simulink model "inflowMatrix"  (R2018a)
settings: Solver=ode1  StartTime=0.0  StopTime=5  FixedStep=1/100  RelTol=1e-3
values from neighbouring files (symbols this model uses):
  s = (0.70:0.02:2.80)    [fy.m]
undefined symbols (not defined in the file or in its folder): deg, rad
libraries: aerolibconvert2 x6
settings Model: PauseTimes=25  Creator=ali  LastModifiedBy=ali

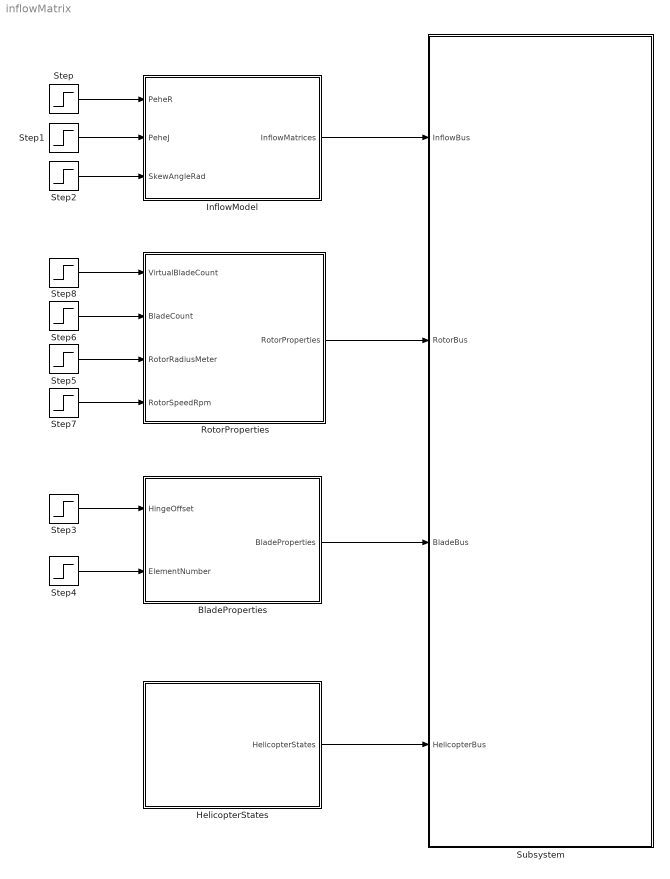
== system inflowMatrix ==
  BladeProperties : Subsystem  TreatAsAtomicUnit=on
  HelicopterStates : Subsystem  TreatAsAtomicUnit=on
  InflowModel : Subsystem  TreatAsAtomicUnit=on
  RotorProperties : Subsystem  TreatAsAtomicUnit=on
  Step : Step  Time=25  Before=2  After=4  SampleTime=0
  Step1 : Step  Time=25  Before=4  After=4  SampleTime=0
  Step2 : Step  Time=0.5  Before=0.0 * pi / 180  After=0.0 * pi / 180  SampleTime=0
  Step3 : Step  Time=0.5  Before=0.01  After=0.01  SampleTime=0
  Step4 : Step  Time=0.5  Before=10  After=10  SampleTime=0
  Step5 : Step  Time=0.5  Before=6  After=6  SampleTime=0
  Step6 : Step  Time=0.5  Before=4  After=4  SampleTime=0
  Step7 : Step  Time=0.5  Before=300  After=300  SampleTime=0
  Step8 : Step  Time=0.5  Before=8  After=8  SampleTime=0
  Subsystem : Subsystem  TreatAsAtomicUnit=on
  wires:
  Step/1 -> InflowModel/1(PeheR)
  Step1/1 -> InflowModel/2(PeheJ)
  Step2/1 -> InflowModel/3(SkewAngleRad)
  Step3/1 -> BladeProperties/1(HingeOffset)
  Step4/1 -> BladeProperties/2(ElementNumber)
  Step5/1 -> RotorProperties/3(RotorRadiusMeter)
  Step6/1 -> RotorProperties/2(BladeCount)
  Step7/1 -> RotorProperties/4(RotorSpeedRpm)
  RotorProperties/1(RotorProperties) -> Subsystem/2(RotorBus)
  BladeProperties/1(BladeProperties) -> Subsystem/3(BladeBus)
  InflowModel/1(InflowMatrices) -> Subsystem/1(InflowBus)
  HelicopterStates/1(HelicopterStates) -> Subsystem/4(HelicopterBus)
  Step8/1 -> RotorProperties/1(VirtualBladeCount)

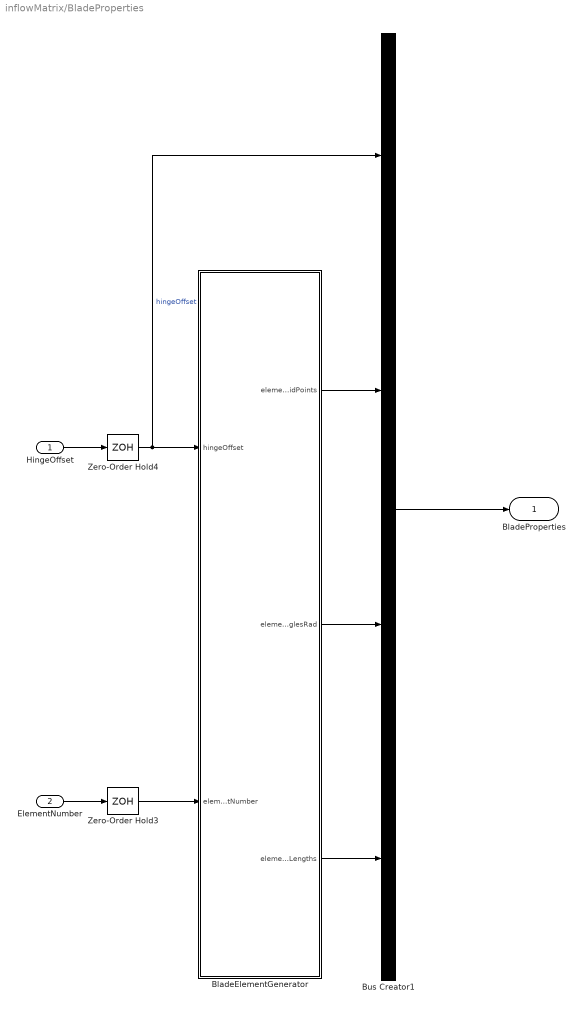
== system inflowMatrix/BladeProperties ==
  HingeOffset : Inport  OutDataTypeStr=double
  ElementNumber : Inport  Port=2  OutDataTypeStr=double
  BladeElementGenerator : MATLAB Function  TreatAsAtomicUnit=on
  Bus Creator1 : BusCreator  Inputs=4
  Zero-Order Hold3 : ZeroOrderHold  SampleTime=-1
  Zero-Order Hold4 : ZeroOrderHold  SampleTime=-1
  BladeProperties : Outport
  wires:
  Zero-Order Hold3/1 -> BladeElementGenerator/2(elementNumber)
  Zero-Order Hold4/1 -> Bus Creator1/1, BladeElementGenerator/1(hingeOffset)  "hingeOffset"
  HingeOffset/1 -> Zero-Order Hold4/1
  ElementNumber/1 -> Zero-Order Hold3/1
  Bus Creator1/1 -> BladeProperties/1
  BladeElementGenerator/1(elementMidPoints) -> Bus Creator1/2
  BladeElementGenerator/2(elementTwistAnglesRad) -> Bus Creator1/3
  BladeElementGenerator/3(elementChordLengths) -> Bus Creator1/4

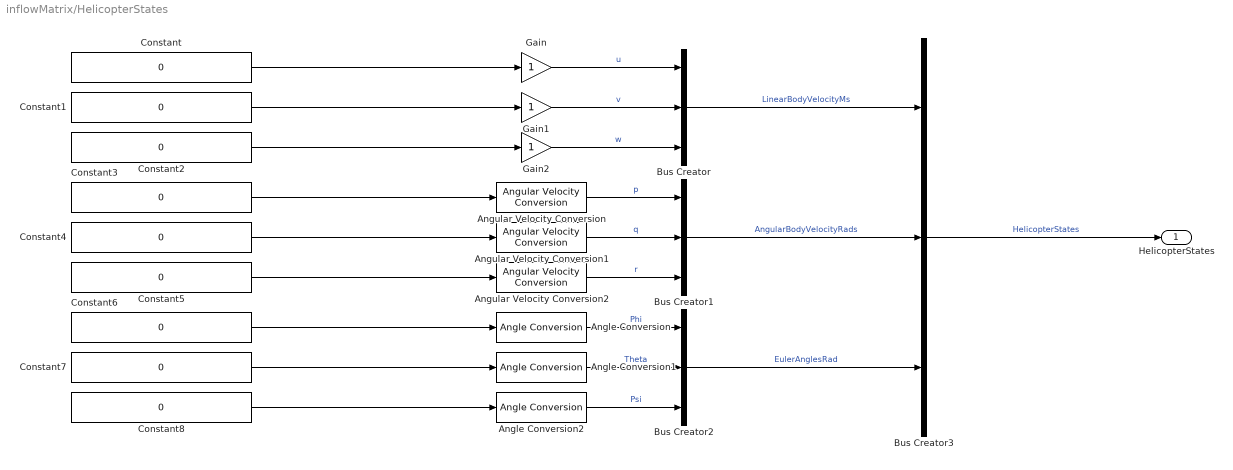
== system inflowMatrix/HelicopterStates ==
  Angle Conversion : aerolibconvert2/Angle Conversion  IU=deg  OU=rad
  Angle Conversion1 : aerolibconvert2/Angle Conversion  IU=deg  OU=rad
  Angle Conversion2 : aerolibconvert2/Angle Conversion  IU=deg  OU=rad
  Angular Velocity Conversion : aerolibconvert2/Angular Velocity Conversion  IU=deg/s  OU=rad/s
      settings: SourceProductName=Aerospace Blockset
  Angular Velocity Conversion1 : aerolibconvert2/Angular Velocity Conversion  IU=deg/s  OU=rad/s
      settings: SourceProductName=Aerospace Blockset
  Angular Velocity Conversion2 : aerolibconvert2/Angular Velocity Conversion  IU=deg/s  OU=rad/s
      settings: SourceProductName=Aerospace Blockset
  Bus Creator{,1..3} (4 alike) : BusCreator  Inputs=3
  Constant{,1..8} (9 alike) : Constant  Value=0
  Gain : Gain
  Gain1 : Gain
  Gain2 : Gain
  HelicopterStates : Outport
  wires:
  Bus Creator/1 -> Bus Creator3/1  "LinearBodyVelocityMs"
  Constant/1 -> Gain/1
  Constant1/1 -> Gain1/1
  Constant2/1 -> Gain2/1
  Gain/1 -> Bus Creator/1  "u"
  Gain1/1 -> Bus Creator/2  "v"
  Gain2/1 -> Bus Creator/3  "w"
  Constant3/1 -> Angular Velocity Conversion/1
  Constant4/1 -> Angular Velocity Conversion1/1
  Constant5/1 -> Angular Velocity Conversion2/1
  Angular Velocity Conversion/1 -> Bus Creator1/1  "p"
  Angular Velocity Conversion1/1 -> Bus Creator1/2  "q"
  Angular Velocity Conversion2/1 -> Bus Creator1/3  "r"
  Constant6/1 -> Angle Conversion/1
  Constant7/1 -> Angle Conversion1/1
  Constant8/1 -> Angle Conversion2/1
  Angle Conversion/1 -> Bus Creator2/1  "Phi"
  Angle Conversion1/1 -> Bus Creator2/2  "Theta"
  Angle Conversion2/1 -> Bus Creator2/3  "Psi"
  Bus Creator1/1 -> Bus Creator3/2  "AngularBodyVelocityRads"
  Bus Creator2/1 -> Bus Creator3/3  "EulerAnglesRad"
  Bus Creator3/1 -> HelicopterStates/1  "HelicopterStates"

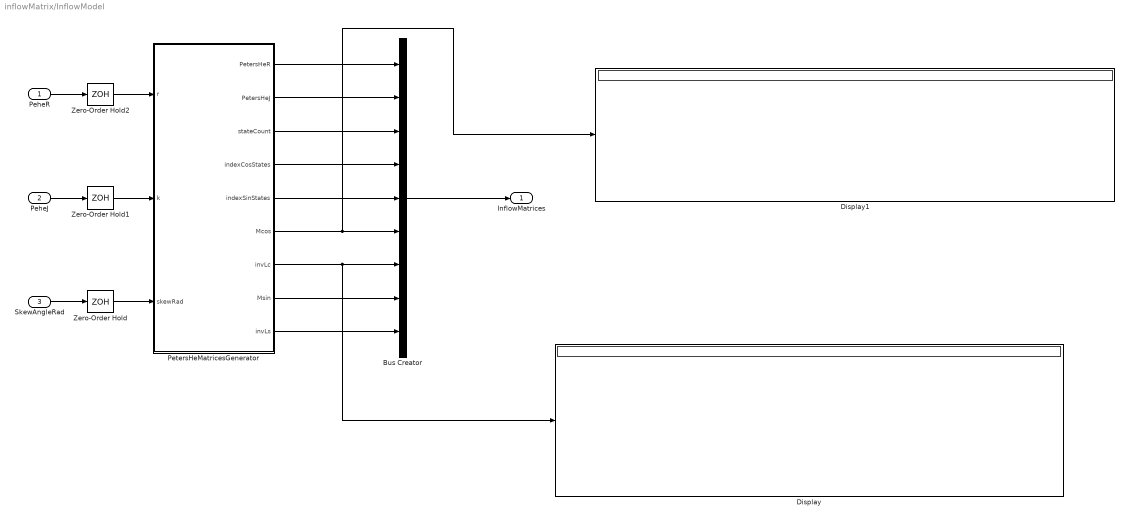
== system inflowMatrix/InflowModel ==
  PeheR : Inport
  PeheJ : Inport  Port=2
  SkewAngleRad : Inport  Port=3
  Bus Creator : BusCreator  Inputs=9
  Display : Display
  Display1 : Display
  PetersHeMatricesGenerator : MATLAB Function  TreatAsAtomicUnit=on
  Zero-Order Hold : ZeroOrderHold  SampleTime=-1
  Zero-Order Hold1 : ZeroOrderHold  SampleTime=-1
  Zero-Order Hold2 : ZeroOrderHold  SampleTime=-1
  InflowMatrices : Outport
  wires:
  Zero-Order Hold1/1 -> PetersHeMatricesGenerator/2(k)
  Zero-Order Hold/1 -> PetersHeMatricesGenerator/3(skewRad)
  PeheR/1 -> Zero-Order Hold2/1
  SkewAngleRad/1 -> Zero-Order Hold/1
  Zero-Order Hold2/1 -> PetersHeMatricesGenerator/1(r)
  PeheJ/1 -> Zero-Order Hold1/1
  PetersHeMatricesGenerator/4(indexCosStates) -> Bus Creator/4
  PetersHeMatricesGenerator/5(indexSinStates) -> Bus Creator/5
  PetersHeMatricesGenerator/6(Mcos) -> Display1/1, Bus Creator/6
  PetersHeMatricesGenerator/7(invLc) -> Display/1, Bus Creator/7
  PetersHeMatricesGenerator/8(Msin) -> Bus Creator/8
  PetersHeMatricesGenerator/9(invLs) -> Bus Creator/9
  PetersHeMatricesGenerator/3(stateCount) -> Bus Creator/3
  PetersHeMatricesGenerator/1(PetersHeR) -> Bus Creator/1
  PetersHeMatricesGenerator/2(PetersHeJ) -> Bus Creator/2
  Bus Creator/1 -> InflowMatrices/1

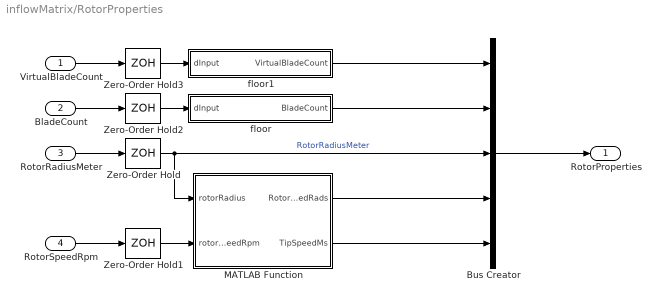
== system inflowMatrix/RotorProperties ==
  VirtualBladeCount : Inport  OutDataTypeStr=double
  BladeCount : Inport  Port=2  OutDataTypeStr=double
  RotorRadiusMeter : Inport  Port=3  OutDataTypeStr=double
  RotorSpeedRpm : Inport  Port=4  OutDataTypeStr=double
  Bus Creator : BusCreator  Inputs=5
  MATLAB Function : MATLAB Function  TreatAsAtomicUnit=on
  Zero-Order Hold{,1..3} (4 alike) : ZeroOrderHold  SampleTime=-1
  floor : MATLAB Function  TreatAsAtomicUnit=on
  floor1 : MATLAB Function  TreatAsAtomicUnit=on
  RotorProperties : Outport
  wires:
  RotorSpeedRpm/1 -> Zero-Order Hold1/1
  MATLAB Function/1(RotorSpeedRads) -> Bus Creator/4
  RotorRadiusMeter/1 -> Zero-Order Hold/1
  MATLAB Function/2(TipSpeedMs) -> Bus Creator/5
  Bus Creator/1 -> RotorProperties/1
  BladeCount/1 -> Zero-Order Hold2/1
  floor/1(BladeCount) -> Bus Creator/2
  Zero-Order Hold/1 -> Bus Creator/3, MATLAB Function/1(rotorRadius)  "RotorRadiusMeter"
  Zero-Order Hold2/1 -> floor/1(dInput)
  Zero-Order Hold1/1 -> MATLAB Function/2(rotorSpeedRpm)
  VirtualBladeCount/1 -> Zero-Order Hold3/1
  Zero-Order Hold3/1 -> floor1/1(dInput)
  floor1/1(VirtualBladeCount) -> Bus Creator/1

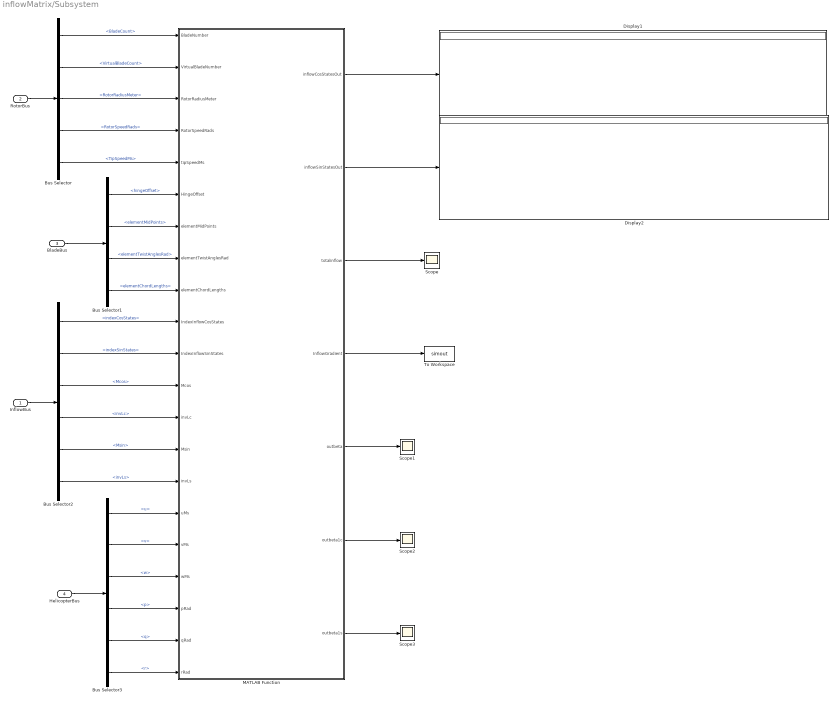
== system inflowMatrix/Subsystem ==
  InflowBus : Inport
  RotorBus : Inport  Port=2
  BladeBus : Inport  Port=3
  HelicopterBus : Inport  Port=4
  Bus Selector : BusSelector  OutputSignals=BladeCount,VirtualBladeCount,RotorRadiusMeter,RotorSpeedRads,TipSpeedMs
  Bus Selector1 : BusSelector  OutputSignals=hingeOffset,elementMidPoints,elementTwistAnglesRad,elementChordLengths
  Bus Selector2 : BusSelector  OutputSignals=indexCosStates,indexSinStates,Mcos,invLc,Msin,invLs
  Bus Selector3 : BusSelector  OutputSignals=LinearBodyVelocityMs.u,LinearBodyVelocityMs.v,LinearBodyVelocityMs.w,AngularBodyVelocityRads.p,AngularBodyVelocityRads.q,AngularBodyVelocityRads.r
  Display1 : Display
  Display2 : Display
  MATLAB Function : MATLAB Function  TreatAsAtomicUnit=on
  Scope{,1..3} (4 alike) : Scope
  To Workspace : ToWorkspace  VariableName=simout  SaveFormat=Structure With Time  SampleTime=-1
  wires:
  BladeBus/1 -> Bus Selector1/1
  Bus Selector1/4 -> MATLAB Function/9(elementChordLengths)  "<elementChordLengths>"
  Bus Selector/4 -> MATLAB Function/4(RotorSpeedRads)  "<RotorSpeedRads>"
  Bus Selector/5 -> MATLAB Function/5(tipSpeedMs)  "<TipSpeedMs>"
  Bus Selector/3 -> MATLAB Function/3(RotorRadiusMeter)  "<RotorRadiusMeter>"
  Bus Selector1/2 -> MATLAB Function/7(elementMidPoints)  "<elementMidPoints>"
  Bus Selector1/3 -> MATLAB Function/8(elementTwistAnglesRad)  "<elementTwistAnglesRad>"
  RotorBus/1 -> Bus Selector/1
  InflowBus/1 -> Bus Selector2/1
  MATLAB Function/1(inflowCosStatesOut) -> Display1/1
  Bus Selector2/1 -> MATLAB Function/10(IndexInflowCosStates)  "<indexCosStates>"
  Bus Selector2/2 -> MATLAB Function/11(IndexInflowSinStates)  "<indexSinStates>"
  MATLAB Function/2(inflowSinStatesOut) -> Display2/1
  Bus Selector2/3 -> MATLAB Function/12(Mcos)  "<Mcos>"
  Bus Selector2/4 -> MATLAB Function/13(invLc)  "<invLc>"
  Bus Selector2/5 -> MATLAB Function/14(Msin)  "<Msin>"
  Bus Selector2/6 -> MATLAB Function/15(invLs)  "<invLs>"
  HelicopterBus/1 -> Bus Selector3/1
  Bus Selector3/1 -> MATLAB Function/16(uMs)  "<u>"
  Bus Selector3/2 -> MATLAB Function/17(vMs)  "<v>"
  Bus Selector3/3 -> MATLAB Function/18(wMs)  "<w>"
  Bus Selector3/4 -> MATLAB Function/19(pRad)  "<p>"
  Bus Selector3/5 -> MATLAB Function/20(qRad)  "<q>"
  Bus Selector3/6 -> MATLAB Function/21(rRad)  "<r>"
  Bus Selector1/1 -> MATLAB Function/6(HingeOffset)  "<hingeOffset>"
  Bus Selector/1 -> MATLAB Function/1(BladeNumber)  "<BladeCount>"
  MATLAB Function/3(totalinflow) -> Scope/1
  Bus Selector/2 -> MATLAB Function/2(VirtualBladeNumber)  "<VirtualBladeCount>"
  MATLAB Function/4(InflowGradient) -> To Workspace/1
  MATLAB Function/5(outbeta) -> Scope1/1
  MATLAB Function/6(outbeta1c) -> Scope2/1
  MATLAB Function/7(outbeta1s) -> Scope3/1

== matlab function inflowMatrix/BladeProperties/BladeElementGenerator ==
  data: hingeOffset input double; elementNumber input double; elementMidPoints output double size=400; elementTwistAnglesRad output double size=400; elementChordLengths output double size=400
function [elementMidPoints,elementTwistAnglesRad,elementChordLengths] = fcn(hingeOffset,elementNumber)

[elementMidPoints]         = readElementNumber(hingeOffset,floor(elementNumber));
[elementTwistAnglesRad]    = readTwist(elementMidPoints);
[elementChordLengths]      = readChord(elementMidPoints);

== matlab function inflowMatrix/InflowModel/PetersHeMatricesGenerator ==
  data: PetersHeR output double; PetersHeJ output double; stateCount output double; indexCosStates output double size=60,2; indexSinStates output double size=60,2; r input double; Mcos output double size=60,60; k input double; skewRad input double; invLc output double size=60,60; Msin output double size=60,60; invLs output double size=60,60
function [PetersHeR,PetersHeJ, stateCount,indexCosStates,indexSinStates,Mcos,invLc,Msin,invLs] = fcn(r,k,skewRad)
 PetersHeR = floor(r);
 PetersHeJ = floor(k);
[stateCount,indexCosStates,indexSinStates,Mcos,invLc,Msin,invLs] = CreateInflowMatrices(PetersHeR,PetersHeJ,skewRad);

== matlab function inflowMatrix/Subsystem/MATLAB Function ==
  data: BladeNumber input double; VirtualBladeNumber input double; RotorRadiusMeter input double; RotorSpeedRads input double; tipSpeedMs input double; HingeOffset input double; inflowCosStatesOut output double; elementMidPoints input double size=400; elementTwistAnglesRad input double size=400; elementChordLengths input double size=400; inflowSinStatesOut output double; IndexInflowCosStates input double size=60,2; IndexInflowSinStates input double size=60,2; Mcos input double size=60,60; invLc input double size=60,60; Msin input double size=60,60; invLs input double size=60,60; uMs input double; vMs input double; wMs input double; pRad input double; qRad input double; rRad input double; totalinflow output double; InflowGradient output double size=36,50; outbeta output; outbeta1c output; outbeta1s output
function [inflowCosStatesOut, inflowSinStatesOut,totalinflow, InflowGradient, outbeta, outbeta1c, outbeta1s] = fcn(BladeNumber, VirtualBladeNumber, RotorRadiusMeter, RotorSpeedRads, tipSpeedMs, HingeOffset, elementMidPoints, elementTwistAnglesRad, elementChordLengths,IndexInflowCosStates, IndexInflowSinStates,Mcos,invLc,Msin,invLs, uMs, vMs, wMs, pRad,qRad,rRad)
dt = 0.01;
%Blade Struct
massPerLength = 20.0 ; %kg/m -> assumtion
Params.densityKgm3 = 1.225;
Control.Theta0  = 0.24;
Control.Theta1s = 0.0;
Control.Theta1c = 0.0;

[inflowCosStates, inflowSinStates]  = UpdateInflowStates(1,[],[]);

elementNumber    = length(elementMidPoints);
CosForcingVector = zeros(length(IndexInflowCosStates),1);
SinForcingVector = zeros(length(IndexInflowSinStates),1);

meanInflow = 0.0;
[bladeAzimuths] = CalculateBladeAzimuths(VirtualBladeNumber, RotorSpeedRads, dt);
%Get Flap
%Calculate Flap
[Beta0, Beta1c, Beta1s, Beta1cD, Beta1sD] = ...
    flapping(1, [], [], [],[], [], [], [],[],[],[],[],[],[],[],dt);

BladeLift2Hub       = zeros(VirtualBladeNumber, 1);
BladeDrag2Hub       = zeros(VirtualBladeNumber, 1);
InflowGradient      = zeros(VirtualBladeNumber,elementNumber) ;
totalinflow = 0.0;
Beta = 0.0;
BetaDot = 0.0;
meanInflowTotal = 0.0;
InflowGradient = zeros(36,50);
for bladeNo = 1:1:VirtualBladeNumber
    
    BladeLift       = zeros(VirtualBladeNumber, 1);
    BladeDrag       = zeros(VirtualBladeNumber, 1);
    azimuth         = bladeAzimuths(bladeNo);
    [Beta, BetaDot] = GetAzimuthFlapping(Beta0, Beta1c, Beta1s, Beta1cD, Beta1sD , azimuth, RotorSpeedRads);
    
    for index = 1:1:elementNumber
       
        % Inflow of section 
        [sectionInflow, meanInflow] = CalculateElementInflow(IndexInflowCosStates, IndexInflowSinStates, inflowCosStates, inflowSinStates, elementMidPoints(index), azimuth);
        sectionInflowDim = sectionInflow * RotorSpeedRads * RotorRadiusMeter;
        meanInflowTotal = meanInflowTotal + meanInflow;
        % Velocities of Section
        [Utangential,Uperpendicular] = sectionSpeed(elementMidPoints(index),HingeOffset,RotorRadiusMeter,RotorSpeedRads,  uMs, vMs, wMs, pRad,qRad,rRad, azimuth, sectionInflowDim, Beta, BetaDot);
        
        %Angles of Section
        SectionTheta = Control.Theta0 + Control.Theta1s * sin(azimuth) + Control.Theta1c * cos(azimuth);
        AngleOfAttackRad = sectionAngles(Utangential,Uperpendicular,SectionTheta);
        SectionAreaM2 = elementChordLengths(index) * (elementMidPoints(2) - elementMidPoints(1)) * RotorRadiusMeter; 
        totalSpeedMs = sqrt(Utangential * Utangential + Uperpendicular * Uperpendicular);
        
        %TODO get CL and CD
        [dLift] = sectionLift(Params.densityKgm3, totalSpeedMs, SectionAreaM2, AngleOfAttackRad * 6);
        [dDrag] = sectionDrag(Params.densityKgm3, totalSpeedMs, SectionAreaM2, AngleOfAttackRad * 0.4);
        
        %Save for blade
        BladeLift(bladeNo)          =  BladeLift(bladeNo) + dLift;
        BladeDrag(bladeNo)          =  BladeDrag(bladeNo) + dDrag;
        
        [dCosForcingVector, dSinForcingVector] = CalculatePeheForcingVectors(dLift, IndexInflowCosStates, IndexInflowSinStates ,elementMidPoints(index),RotorRadiusMeter, RotorSpeedRads, Params.densityKgm3);
        CosForcingVector = CosForcingVector + dCosForcingVector;
        SinForcingVector = SinForcingVector + dSinForcingVector; 
        totalinflow = totalinflow + sectionInflowDim * sectionInflowDim * SectionAreaM2 *  Params.densityKgm3;
        InflowGradient(bladeNo,index) = sectionInflowDim;
        
    end
        
end
MeanChordM = 1.5;
MeanClAlpha = 6.0;
%overall Mean Infliow
meanInflowTotal = meanInflowTotal / (VirtualBladeNumber * elementNumber);
%Calculate Flap
[~, ~, ~, ~, ~] = ...
    flapping(2, Control.Theta0, Control.Theta1c, Control.Theta1s, ...
    RotorRadiusMeter,RotorSpeedRads, MeanChordM, MeanClAlpha, Params.densityKgm3,...
    meanInflowTotal, HingeOffset, massPerLength,uMs,vMs,wMs,dt);

CosForcingVector = (CosForcingVector / VirtualBladeNumber) * BladeNumber;
SinForcingVector = (SinForcingVector / VirtualBladeNumber) * BladeNumber;
[CosStatesOut, SinStatesOut] = solveInflow(Mcos,invLc,Msin,invLs,CosForcingVector, SinForcingVector, IndexInflowCosStates,IndexInflowSinStates,uMs,vMs,wMs, meanInflow, tipSpeedMs,RotorSpeedRads, dt);
  
inflowCosStatesOut = CosStatesOut;
inflowSinStatesOut = SinStatesOut;
totalinflow = (totalinflow / VirtualBladeNumber) * BladeNumber;
outbeta = Beta0;
outbeta1c = Beta1c;
outbeta1s = Beta1s;
end

function [inflowCosStates, inflowSinStates] = UpdateInflowStates(GetOrSet, inputCosStates, inputSinStates)
%Initialize and update inflow states % arg = 1 Gets the number, arg = not 1
%updates the states
persistent InflowCosineStates;
if isempty(InflowCosineStates)
    InflowCosineStates = zeros(10,10);
end

persistent InflowSineStates;
if isempty(InflowSineStates)
    InflowSineStates = zeros(10,10);
end
% InflowCosineStates = InflowCosineStates + 0.001;
% InflowSineStates = InflowSineStates + 0.001;
if(1 == GetOrSet)
    inflowCosStates = InflowCosineStates;
    inflowSinStates = InflowSineStates;
elseif(2 == GetOrSet)
    InflowCosineStates = inputCosStates;
    InflowSineStates   = inputSinStates;
    inflowCosStates = InflowCosineStates;
    inflowSinStates = InflowSineStates;
end
end

function [sectionInflow,meanInflow] = CalculateElementInflow(IndexCosStates, IndexSinStates, InflowCosStates, InflowSinStates, rbar, azimuth)
%Calculate inflow using pehe states
% Predetermine variable sizes for output signal size allocation
cosStatesCount = length(IndexCosStates);
sinStatesCount = length(IndexSinStates);
sectionInflow = 0.0;

meanInflow = sectionInflow;

for index = 1:1:cosStatesCount
    % State r and j
    peheR = IndexCosStates(index,1);
    peheJ = IndexCosStates(index,2);
    
    %RadialShapeFunction
    RadialShapeMultiplier = RadialShapeFunc(peheR, peheJ, rbar);
    
    % While Calling InflowCosStates the row number needs to be shifted
    % once, because the index of state starts at 0 but matlab matrix starts
    % a 1. Meaning that state: a03->(r = 0 , j = 3) located at cosStates(1,3)
    % further explanation: at Row zero lies the r=0 state row.
    sectionInflow = sectionInflow +  InflowCosStates(peheR+1,peheJ) * RadialShapeMultiplier * cos(peheR * azimuth);
    if(peheR < 0.5)
        meanInflow = meanInflow +  InflowCosStates(peheR+1,peheJ) * RadialShapeMultiplier * cos(peheR * azimuth);
    end
    
end

for index = 1:1:sinStatesCount
    % State r and j
    peheR = IndexSinStates(index,1);
    peheJ = IndexSinStates(index,2);
    
    %RadialShapeFunction
    RadialShapeMultiplier = RadialShapeFunc(peheR, peheJ, rbar);
    
    %Inflow Contribution
    sectionInflow = sectionInflow + InflowSinStates(peheR,peheJ) * RadialShapeMultiplier * sin(peheR * azimuth) ;
end

end

function [CosStatesOut, SinStatesOut] = solveInflow(Mcos,invLc,Msin,invLs,CosForcingVector, SinForcingVector, indexCosStates,indexSinStates,uMs,vMs,wMs, meanInflow, tipSpeedMs, RotorSpeedRads, dt)
[VCos,Vsin] = FlowMatrix(indexCosStates,indexSinStates,uMs,vMs,wMs, meanInflow, tipSpeedMs);
[CosStates,SinStates] = UpdateInflowStates(1, [], []);

% Get Related States Cos
CosStateCount  = length(indexCosStates);
cosStateVector = zeros(CosStateCount,1);
for index = 1:1:length(indexCosStates)
    cosStateVector(index) = CosStates(indexCosStates(index,1) + 1,indexCosStates(index,2));
end

% Get Related States Sin
SinStateCount  = length(indexSinStates);
sinStateVector = zeros(SinStateCount,1);
for index = 1:1:length(indexSinStates)
    sinStateVector(index) = SinStates(indexSinStates(index,1),indexSinStates(index,2));
end

% invMcos = inv(Mcos);
% invMsin = inv(Msin);

CosStatesDerivatives = Mcos\(0.5 * CosForcingVector - (invLc * VCos) * cosStateVector);
SinStatesDerivatives = Msin\ (0.5 * SinForcingVector - (invLs * Vsin) * sinStateVector);
%
%Integrate States using euler integration and dt = 1/100;
cosStateVector = cosStateVector + dt *  CosStatesDerivatives * RotorSpeedRads * 0.1;
sinStateVector = sinStateVector + dt *  SinStatesDerivatives * RotorSpeedRads * 0.1;
%Place Into State Matrix
for index = 1:1:length(indexCosStates)
    CosStates(indexCosStates(index,1) + 1,indexCosStates(index,2)) = cosStateVector(index);
end
for index = 1:1:length(indexSinStates)
    SinStates(indexSinStates(index,1),indexSinStates(index,2)) = sinStateVector(index);
end
[~,~] = UpdateInflowStates(2, CosStates, SinStates);
CosStatesOut = CosStates;
SinStatesOut = SinStates;
end


function [CosForcingVector, SinForcingVector] = CalculatePeheForcingVectors(dLift, indexCosStates, indexSinStates ,rbar,RotorRadiusMeter, RotorSpeedRads, DensityKgm3)

NonDimensionalizingTerm = pi * DensityKgm3 * RotorSpeedRads * RotorSpeedRads * RotorRadiusMeter * RotorRadiusMeter *RotorRadiusMeter * RotorRadiusMeter;
cosStatesCount = length(indexCosStates);
sinStatesCount = length(indexSinStates);
cosRadialShapeMultiplier = zeros(cosStatesCount,1);
sinRadialShapeMultiplier = zeros(sinStatesCount,1);

for index = 1:1:cosStatesCount
    % State r and j
    peheR = indexCosStates(index,1);
    peheJ = indexCosStates(index,2);
    
    %RadialShapeFunction
    cosRadialShapeMultiplier(index) = RadialShapeFunc(peheR, peheJ, rbar);
   
end
CosForcingVector = cosRadialShapeMultiplier * dLift / NonDimensionalizingTerm;
for index = 1:1:sinStatesCount
    % State r and j
    peheR = indexSinStates(index,1);
    peheJ = indexSinStates(index,2);
    
    %RadialShapeFunction
    sinRadialShapeMultiplier(index) = RadialShapeFunc(peheR, peheJ, rbar);

end
SinForcingVector = sinRadialShapeMultiplier * dLift / NonDimensionalizingTerm;
end

function [bladeAzimuths] = CalculateBladeAzimuths(BladeNumber, RotorSpeedRads, dt)
persistent BladeAzimuthPersist;
if(isempty(BladeAzimuthPersist))
    firstBladeAzimuth = 0.0;
    angleBetweenBlades = 2 * pi/BladeNumber;
    lastBladeAzimuth = 2 * pi - angleBetweenBlades;
    BladeAzimuthPersist = [firstBladeAzimuth:angleBetweenBlades:lastBladeAzimuth];

end

%BladeAzimuthPersist = BladeAzimuthPersist + RotorSpeedRads * dt;

if(BladeAzimuthPersist > 2 * pi)
    BladeAzimuthPersist = BladeAzimuthPersist - 2 * pi;
end

bladeAzimuths = BladeAzimuthPersist;
end

function [Beta, BetaDot] = GetAzimuthFlapping(inBeta0, inBeta1c, inBeta1s, inBeta1cD, inBeta1sD , azimuth, RotorSpeedRads)
Beta = inBeta0 + inBeta1c * cos(azimuth) + inBeta1s * sin(azimuth);
BetaDot = inBeta1cD * cos(azimuth) - RotorSpeedRads*sin(azimuth)*inBeta1c + inBeta1sD*sin(azimuth) + RotorSpeedRads*cos(azimuth)*inBeta1s;
end

== matlab function inflowMatrix/RotorProperties/MATLAB Function ==
  data: rotorRadius input double size=1; RotorSpeedRads output double size=1; rotorSpeedRpm input double size=1; TipSpeedMs output double size=1
function [RotorSpeedRads, TipSpeedMs] = fcn(rotorRadius, rotorSpeedRpm)

RotorSpeedRads = (rotorSpeedRpm / 60.0) * 2.0 * pi;
TipSpeedMs = RotorSpeedRads * rotorRadius;

== matlab function inflowMatrix/RotorProperties/floor ==
  data: dInput input double size=1; BladeCount output double size=1
function BladeCount  = fcn(dInput)
BladeCount = floor(dInput);

== matlab function inflowMatrix/RotorProperties/floor1 ==
  data: dInput input double size=1; VirtualBladeCount output double size=1
function VirtualBladeCount  = fcn(dInput)
VirtualBladeCount = floor(dInput);
